simulink model "frdm_steering_servo"  (R2017a)
settings: Solver=VariableStepAuto  StartTime=0.0  StopTime=inf  RelTol=1e-3
libraries: frdmtfcshieldlib x1
settings Model: SimulationMode=external  Creator=WARA  LastModifiedBy=WARA

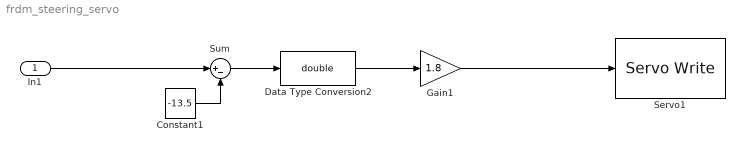
== system frdm_steering_servo ==
  In1 : Inport
  Constant1 : Constant  Value=-13.5
  Data Type Conversion2 : DataTypeConversion  OutDataTypeStr=double
  Gain1 : Gain  Gain=1.8
  Servo1 : frdmtfcshieldlib/Servo Write  WhichServo=0  minAngle=-30  maxAngle=70
      settings: SourceProductName=Simulink Coder Support Package for NXP FRDM-KL25Z Board  SourceProductBaseCode=EC_FREEDOM_BOARD
  Sum : Sum  Inputs=|+-
  wires:
  Data Type Conversion2/1 -> Gain1/1
  Constant1/1 -> Sum/2
  Gain1/1 -> Servo1/1
  Sum/1 -> Data Type Conversion2/1
  In1/1 -> Sum/1
